simulink model "Torque_Converter_control"  (Simulink 8.2)
settings: Solver=ode45  StartTime=0.0  StopTime=10.0  RelTol=1e-3
model workspace (MAT data in the model file):
  min_gear_number_thresh = Simulink.Parameter
  min_gear_number_thresh.Value = 4
  min_gear_number_thresh.DataType = 'int32'
  min_speed_ratio_thresh = Simulink.Parameter
  min_speed_ratio_thresh.Value = 0.925
  min_speed_ratio_thresh.DataType = 'double'
  pedal_disable_thresh = Simulink.Parameter
  pedal_disable_thresh.Value = 0.85
  pedal_disable_thresh.DataType = 'double'
  pedal_enable_thresh = Simulink.Parameter
  pedal_enable_thresh.Value = 0.8415
  pedal_enable_thresh.DataType = 'double'
settings Model: Creator=jporter  LastModifiedBy=tiwari
settings DebuggingCC: FcnCallInpInsideContextMsg=EnableAllAsWarning
settings GRTTargetCC: CombineOutputUpdateFcns=on  GRTInterface=off

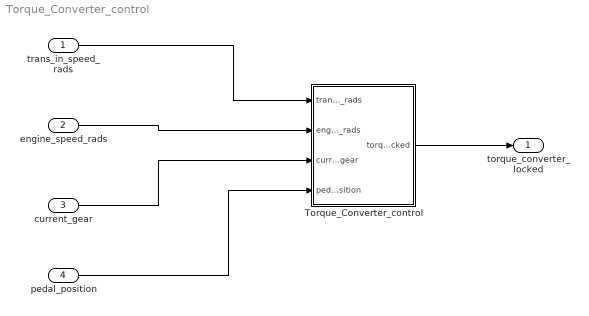
== system Torque_Converter_control ==
  trans_in_speed_rads : Inport  OutDataTypeStr=double
  engine_speed_rads : Inport  Port=2  OutDataTypeStr=double
  current_gear : Inport  Port=3  OutDataTypeStr=int32
  pedal_position : Inport  Port=4  OutDataTypeStr=double
  Torque_Converter_control : Subsystem
  torque_converter_locked : Outport  OutDataTypeStr=double
  wires:
  trans_in_speed_rads/1 -> Torque_Converter_control/1(trans_in_speed_rads)
  engine_speed_rads/1 -> Torque_Converter_control/2(engine_speed_rads)
  current_gear/1 -> Torque_Converter_control/3(current_gear)
  pedal_position/1 -> Torque_Converter_control/4(pedal_position)
  Torque_Converter_control/1(torque_converter_locked) -> torque_converter_locked/1

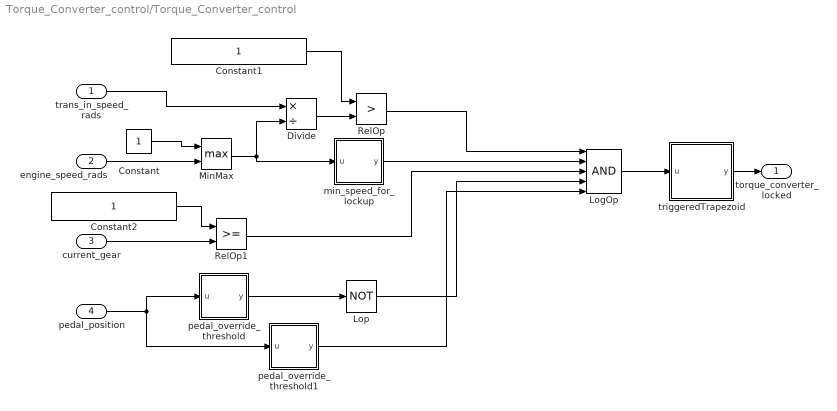
== system Torque_Converter_control/Torque_Converter_control ==
  trans_in_speed_rads : Inport  OutDataTypeStr=double
  engine_speed_rads : Inport  Port=2  OutDataTypeStr=double
  current_gear : Inport  Port=3  OutDataTypeStr=int32
  pedal_position : Inport  Port=4  OutDataTypeStr=double
  Constant : Constant
  Constant1 : Constant
  Constant2 : Constant
  Divide : Product  Inputs=*/
  LogOp : Logic  Inputs=5  AllPortsSameDT=off  OutDataTypeStr=boolean
  Lop : Logic  Operator=NOT  AllPortsSameDT=off  OutDataTypeStr=boolean
  MinMax : MinMax  Function=max  Inputs=2
  RelOp : RelationalOperator  Operator=>  OutDataTypeStr=boolean
  RelOp1 : RelationalOperator  OutDataTypeStr=boolean
  min_speed_for_lockup : Subsystem
  pedal_override_threshold : Subsystem
  pedal_override_threshold1 : Subsystem
  triggeredTrapezoid : Stateflow chart  TreatAsAtomicUnit=on
  torque_converter_locked : Outport  OutDataTypeStr=double
  wires:
  Constant/1 -> MinMax/1
  MinMax/1 -> Divide/2, min_speed_for_lockup/1(u)
  Constant1/1 -> RelOp/1
  Divide/1 -> RelOp/2
  RelOp/1 -> LogOp/1
  min_speed_for_lockup/1(y) -> LogOp/2
  Constant2/1 -> RelOp1/1
  RelOp1/1 -> LogOp/3
  pedal_override_threshold/1(y) -> Lop/1
  Lop/1 -> LogOp/4
  pedal_override_threshold1/1(y) -> LogOp/5
  LogOp/1 -> triggeredTrapezoid/1(u)
  triggeredTrapezoid/1(y) -> torque_converter_locked/1
  trans_in_speed_rads/1 -> Divide/1
  engine_speed_rads/1 -> MinMax/2
  current_gear/1 -> RelOp1/2
  pedal_position/1 -> pedal_override_threshold/1(u), pedal_override_threshold1/1(u)

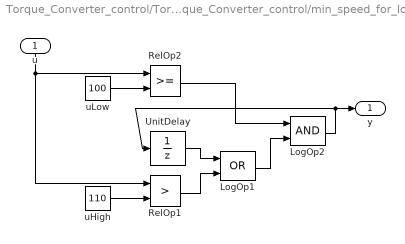
== system Torque_Converter_control/Torque_Converter_control/min_speed_for_lockup ==
  u : Inport
  LogOp1 : Logic  Operator=OR  AllPortsSameDT=off  OutDataTypeStr=boolean
  LogOp2 : Logic  AllPortsSameDT=off  OutDataTypeStr=boolean
  RelOp1 : RelationalOperator  Operator=>  OutDataTypeStr=boolean
  RelOp2 : RelationalOperator  OutDataTypeStr=boolean
  UnitDelay : UnitDelay  SampleTime=-1
  uHigh : Constant  Value=110
  uLow : Constant  Value=100
  y : Outport
  wires:
  UnitDelay/1 -> LogOp1/1
  RelOp1/1 -> LogOp1/2
  uLow/1 -> RelOp2/2
  uHigh/1 -> RelOp1/2
  RelOp2/1 -> LogOp2/1
  LogOp1/1 -> LogOp2/2
  LogOp2/1 -> UnitDelay/1, y/1
  u/1 -> RelOp2/1, RelOp1/1

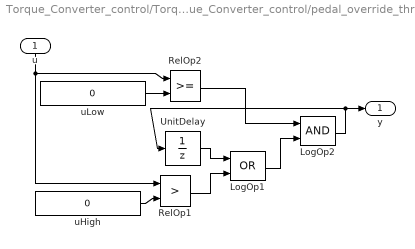
== system Torque_Converter_control/Torque_Converter_control/pedal_override_threshold ==
  u : Inport
  LogOp1 : Logic  Operator=OR  AllPortsSameDT=off  OutDataTypeStr=boolean
  LogOp2 : Logic  AllPortsSameDT=off  OutDataTypeStr=boolean
  RelOp1 : RelationalOperator  Operator=>  OutDataTypeStr=boolean
  RelOp2 : RelationalOperator  OutDataTypeStr=boolean
  UnitDelay : UnitDelay  SampleTime=-1
  uHigh : Constant  Value=0
  uLow : Constant  Value=0
  y : Outport
  wires:
  UnitDelay/1 -> LogOp1/1
  RelOp1/1 -> LogOp1/2
  uLow/1 -> RelOp2/2
  uHigh/1 -> RelOp1/2
  RelOp2/1 -> LogOp2/1
  LogOp1/1 -> LogOp2/2
  LogOp2/1 -> UnitDelay/1, y/1
  u/1 -> RelOp2/1, RelOp1/1

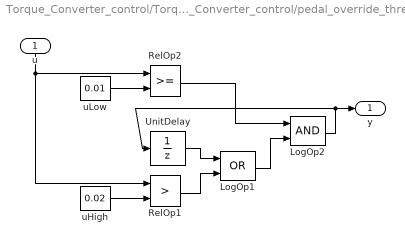
== system Torque_Converter_control/Torque_Converter_control/pedal_override_threshold1 ==
  u : Inport
  LogOp1 : Logic  Operator=OR  AllPortsSameDT=off  OutDataTypeStr=boolean
  LogOp2 : Logic  AllPortsSameDT=off  OutDataTypeStr=boolean
  RelOp1 : RelationalOperator  Operator=>  OutDataTypeStr=boolean
  RelOp2 : RelationalOperator  OutDataTypeStr=boolean
  UnitDelay : UnitDelay  SampleTime=-1
  uHigh : Constant  Value=0.02
  uLow : Constant  Value=0.01
  y : Outport
  wires:
  UnitDelay/1 -> LogOp1/1
  RelOp1/1 -> LogOp1/2
  uLow/1 -> RelOp2/2
  uHigh/1 -> RelOp1/2
  RelOp2/1 -> LogOp2/1
  LogOp1/1 -> LogOp2/2
  LogOp2/1 -> UnitDelay/1, y/1
  u/1 -> RelOp2/1, RelOp1/1

== stateflow chart Torque_Converter_control/triggeredTrapezoid ==
  settings: description=|
      | <?xml version="1.0" encoding="utf-8"?>
      | <ltlProperties AbsenceCount="4">
      |    <ltlProperty afterExpr="" beforeExpr="" expr="[](!((y &lt; 0) || (y &gt; 1)))" id="Absence1" name="AbsenceProperty" rawProperty="(y &lt; 0) || (y &gt; 1)" rawProperty2="" scope="Global" type="Absence"/>
      |    <ltlProperty afterExpr="" beforeExpr="" expr="[](!((y &lt; 0) || (y &gt; 0.4)))" id="Absence2" name="AbsenceProperty1" rawProperty="(y &lt; 0) || (y &gt; 0.4)" rawProperty2="" scope="Global" type="Absence"/>
      |    <ltlProperty afterExpr="" beforeExpr="" expr="[](!((y &lt; 0.1) || (y &gt; 1)))" id="Absence3" name="AbsenceProperty12" rawProperty="(y &lt; 0.1) || (y &gt; 1)" rawProperty2="" scope="Global" type="Absence"/>
      |    <ltlProperty afterExpr="" beforeExpr="" expr="[](!(triggeredTrapezoidMode = Falling))" id="Absence4" name="AbsenceProperty123" rawProperty="triggeredTrapezoidMode = Falling" rawProperty2="" scope="Global" type="Absence"/>
      | </ltlProperties>
  state Low
    entry: y = offset;
  state Rising
    during: y = y + rise_step;
  state Falling
    during: y = y - fall_step;
  state High
    entry: y = amplitude+offset;
  (default) -> Low : / rise_step = amplitude / (rise_time / sample_period);
      |  fall_step = amplitude / (fall_time / sample_period);
  Falling -> Low [order 1] : [y <= offset]
  Low -> Rising : [u == true]
  Rising -> Falling [order 2] : [u==false]
  Falling -> Rising [order 2] : [u==true]
  Rising -> High [order 1] : [y >= amplitude+offset]
  High -> Falling : [u == false]
  data: sample_period local double; u input boolean; amplitude local double =1; rise_time local double =0.2; fall_time local double =0.2; offset local double =0; rise_step local double =0.0; fall_step local double =0.0; y output double =0
